simulink model "mdlkolmogo"  (Simulink 7.8)
settings: Solver=ode45  StartTime=0.0  StopTime=40  RelTol=1e-3
settings Model: Creator=klempond  LastModifiedBy=polacekm
settings GRTTargetCC: CombineOutputUpdateFcns=on

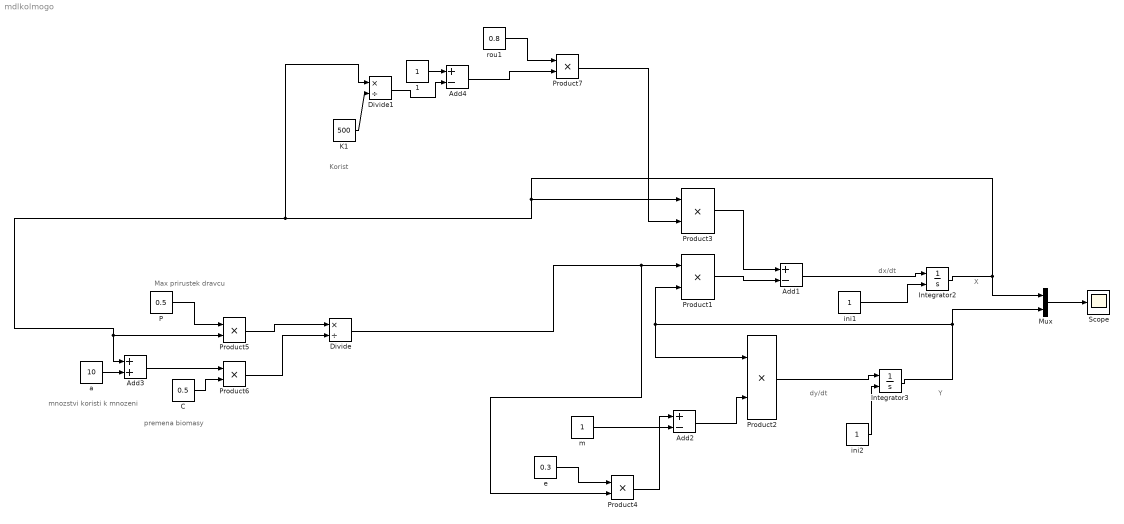
== system mdlkolmogo ==
  note: X
  note: dx/dt
  note: dy/dt
  note: Y
  note: Max prirustek dravcu
  note: mnozstvi koristi k mnozeni
  note: premena biomasy
  note: Korist
  1 : Constant
  Add1 : Sum  Inputs=+-
  Add2 : Sum  Inputs=+-
  Add3 : Sum
  Add4 : Sum  Inputs=+-
  C : Constant  Value=0.5
  Divide : Product  Inputs=*/
  Divide1 : Product  Inputs=*/
  Integrator2 : Integrator  InitialConditionSource=external  InitialCondition=100
  Integrator3 : Integrator  InitialConditionSource=external  InitialCondition=10
  K1 : Constant  Value=500
  Mux : Mux  Inputs=2
  P : Constant  Value=0.5
  Product{1..7} (7 alike) : Product  RndMeth=Zero
  Scope : Scope
      settings: SaveName=sc
  a : Constant  Value=10
  e : Constant  Value=0.3
  ini1 : Constant
  ini2 : Constant
  m : Constant
  rou1 : Constant  Value=0.8
  wires:
  Product2/1 -> Integrator3/1
  Integrator3/1 -> Product2/1, Product1/2, Mux/2
  Add2/1 -> Product2/2
  Product1/1 -> Add1/2
  Product3/1 -> Add1/1
  Add1/1 -> Integrator2/1
  Integrator2/1 -> Product3/1, Add3/1, Product5/2, Divide1/1, Mux/1
  Mux/1 -> Scope/1
  ini2/1 -> Integrator3/2
  ini1/1 -> Integrator2/2
  Product4/1 -> Add2/1
  e/1 -> Product4/1
  m/1 -> Add2/2
  P/1 -> Product5/1
  Divide/1 -> Product1/1, Product4/2
  Product6/1 -> Divide/2
  Product5/1 -> Divide/1
  Add3/1 -> Product6/1
  C/1 -> Product6/2
  a/1 -> Add3/2
  Product7/1 -> Product3/2
  rou1/1 -> Product7/1
  1/1 -> Add4/1
  Divide1/1 -> Add4/2
  K1/1 -> Divide1/2
  Add4/1 -> Product7/2
